simulink model "diagrama2"  (R2025b)
settings: Solver=VariableStepAuto  StartTime=0.0  StopTime=100  RelTol=1e-3
model workspace (MAT data in the model file):
  A1 = 15.518
  A2 = 15.518
  a1 = 0.138
  a2 = 0.419
  g = 981
  gama = 0.5
settings Model: Creator=cafe2  LastModifiedBy=sergioe.ropero

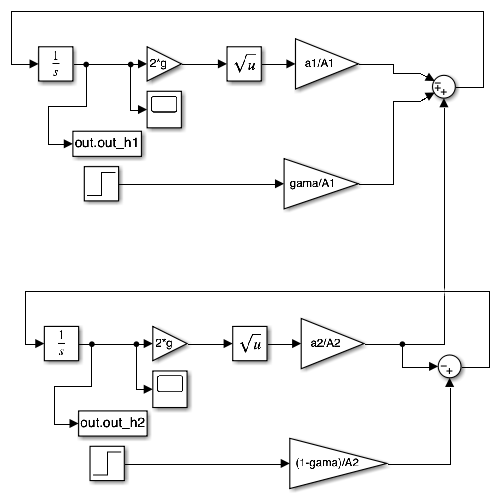
[thumbnail: Simulink's stored preview of the top-level diagram]
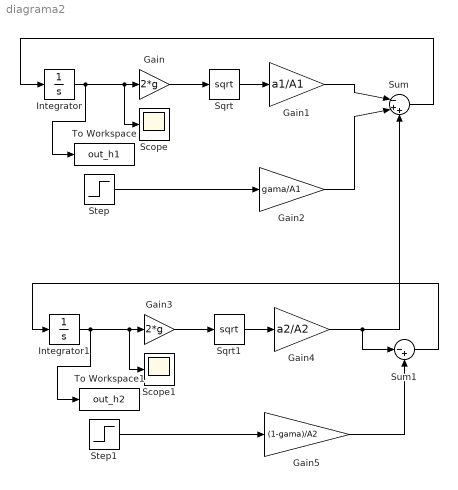
== system diagrama2 ==
  Gain : Gain  Gain=2*g
  Gain1 : Gain  Gain=a1/A1
  Gain2 : Gain  Gain=gama/A1
  Gain3 : Gain  Gain=2*g
  Gain4 : Gain  Gain=a2/A2
  Gain5 : Gain  Gain=(1-gama)/A2
  Integrator : Integrator
  Integrator1 : Integrator
  Scope : Scope
      settings: ActiveDisplayYMinimum=-2.2255706032573817  ActiveDisplayYMaximum=20.030135429316438
  Scope1 : Scope
      settings: ActiveDisplayYMinimum=-0.060811690089787672  ActiveDisplayYMaximum=0.54730521080808914
  Sqrt : Sqrt
  Sqrt1 : Sqrt
  Step : Step  After=25.89
  Step1 : Step  After=25.89
  Sum : Sum  Inputs=|-++
  Sum1 : Sum  Inputs=|-+
  To Workspace : ToWorkspace  VariableName=out_h1  SaveFormat=Timeseries  SampleTime=-1
  To Workspace1 : ToWorkspace  VariableName=out_h2  SaveFormat=Timeseries  SampleTime=-1
  wires:
  Sqrt/1 -> Gain1/1
  Gain/1 -> Sqrt/1
  Gain1/1 -> Sum/1
  Step/1 -> Gain2/1
  Gain2/1 -> Sum/2
  Sum/1 -> Integrator/1
  Integrator/1 -> To Workspace/1, Scope/1, Gain/1
  Sqrt1/1 -> Gain4/1
  Gain5/1 -> Sum1/2
  Step1/1 -> Gain5/1
  Gain4/1 -> Sum/3, Sum1/1
  Integrator1/1 -> To Workspace1/1, Scope1/1, Gain3/1
  Gain3/1 -> Sqrt1/1
  Sum1/1 -> Integrator1/1
